simulink model "eq_sim"  (Simulink 6.0)
settings: Solver=VariableStepDiscrete  SolverMode=SingleTasking  StartTime=0.0  StopTime=10  RelTol=1e-3
StopFcn:
  | % Call to callback function in eq_initmask
  | if exist('taps','var')
  | eq_initmask([gcs '/Initial Settings'],'plotCostTrajectory',taps,tapsRef,eq);
  | end
model workspace: external: M-Code (data not in the file)
values from neighbouring files (symbols this model uses):
  eq = varargin{3}    [eq_initmask.m]
undefined symbols (not defined in the file or in its folder): eq_getopt, eq_mmseconverg, Fs, slcm
libraries: simulink x8, dspsigops x7, dspsrcs4 x6, dspsnks4 x6, commsink2 x5, dspsigattribs x5, commdigbbndam2 x3, commeq2 x2, dspindex x2, dspbuff3 x2, commchan2 x1, dsparch4 x1
CloseFcn:
  | % Call to callback function in eq_initmask
  | eq_initmask([gcs '/Initial Settings'],'CloseFcn');
settings Model: Creator=arodrigu  LastModifiedBy=arodrigu
settings DataIOCC: LimitDataPoints=off  SaveOutput=off  SaveTime=off  SignalLoggingName=eqSigsOut
settings OptimizationCC: BooleanDataType=off  InlineInvariantSignals=off
settings DebuggingCC: CheckExecutionContextPreStartOutputMsg=on  CheckExecutionContextRuntimeOutputMsg=on  SolverPrmCheckMsg=none  InheritedTsInSrcMsg=none
settings HardwareCC: TargetUnknown=on
settings ModelReferenceCC: UpdateModelReferenceTargets=IfOutOfDate
settings CodeAppCC: PrefixModelToSubsysFcnNames=off

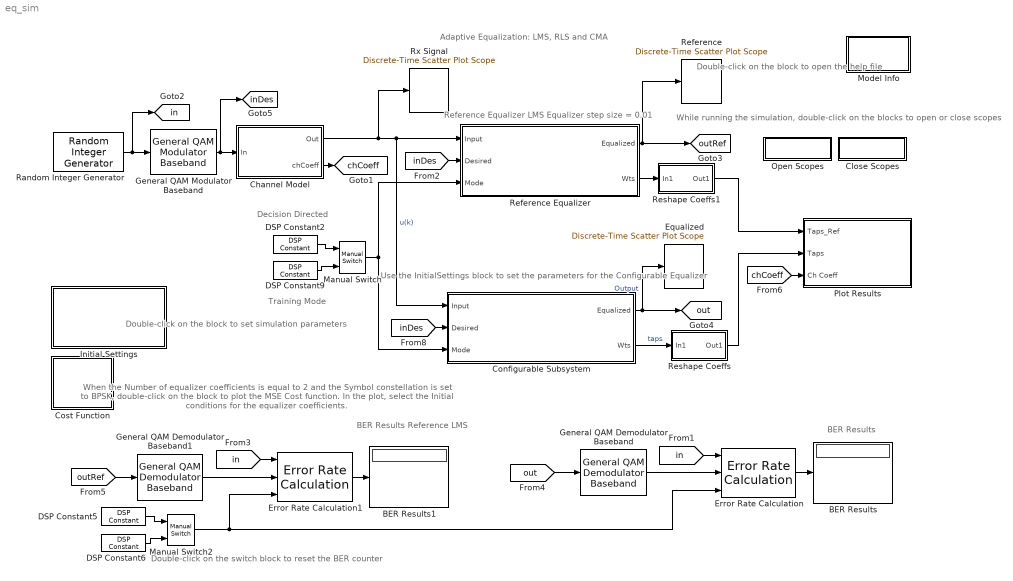
== system eq_sim ==
  note: Adaptive Equalization: LMS, RLS and CMA
  note: When the Number of equalizer coefficients is equal to 2 and the
      | Symbol constellation is set to BPSK, double-click on the block to plot
      | the MSE Cost function. In the plot, select the Initial conditions
      | for the equalizer coefficients.
  note: Double-click on the block
      | to set simulation parameters
  note: While running the simulation,
      | double-click on the blocks
      | to open or close scopes
  note: Training Mode
  note: Decision Directed
  note: BER Results
      | Reference LMS
  note: Double-click on the switch block
      | to reset the BER counter
  note: Reference Equalizer
      | LMS Equalizer
      | step size = 0.01
  note: BER Results
  note: Double-click on the block
      | to open the help file
  note: Use the InitialSettings block
      | to set the parameters for
      | the Configurable Equalizer
  BER Results : Display
  BER Results1 : Display
  Channel Model : Subsystem  PropExecContextAcrossSSBoundary=on  mask(Channel Model){chCoeff=eq.chCoeff, snrdB=eq.snrdB}
      mask prompts: chCoeff "Channel Coefficients:"; snrdB "SNR (in dB):"
      mask init:
      | chCoeff_fdB = 10*log10(abs(abs(fftshift(fft(chCoeff,256)))));
      | sigmaN2 = 10^(-snrdB/10);
      mask Display: plot([-pi:pi/128:(pi-pi/128)],chCoeff_fdB);
  Close Scopes : Subsystem  PropExecContextAcrossSSBoundary=on
      settings: OpenFcn=|
      | str1 = 'Plot Results';
      |         str2 = 'MSE Convergency Plot';
      |         str3 = 'Equalizer Response';
      |         str4 = 'Equalizer Taps - Real';
      |         str5 = 'Equalizer Taps - Imag';
      |         str6 = 'Rx Signal';
      |         str7 = 'Reference';
      |         str8 = 'Equalized';
      | 
      |         sdspfscope2([],[],[],'ScopeUpdate',[bdroot '/' str1 '/' str2 ],'CloseFig');
      |         sdspfscope2([],[],[],'ScopeUpdate',[bdroot '/' str1 '/' str3 ],'CloseFig');
      |         sdspfscope2([],[],[],'ScopeUpdate',[bdroot '/' str1 '/' str4 ],'CloseFig');
      |         sdspfscope2([],[],[],'ScopeUpdate',[bdroot '/' str1 '/' str5 ],'CloseFig');
      | 
      |         sdspfscope2([],[],[],'ScopeUpdate',[bdroot '/' str6 ],'CloseFig');
      |         sdspfscope2([],[],[],'ScopeUpdate',[bdroot '/' str7 ],'CloseFig');
      |         sdspfscope2([],[],[],'ScopeUpdate',[bdroot '/' str8 ],'CloseFig');
      mask Display: disp('Close Scopes');
  Configurable Subsystem : Subsystem  BlockChoice="RLS Linear  Equalizer"  PropExecContextAcrossSSBoundary=on
      link override CMA Equalizer: nTaps=eq.numTaps  sigConst=eq.const  delay=eq.delta_opt+1  stepSize=eq.stepSize  leakage=eq.leakage  initWeights=eq.ic
      link override LMS Linear  Equalizer: nTaps=eq.numTaps  sigConst=eq.const  delay=eq.delta_opt+1  stepSize=eq.stepSize  leakage=eq.leakage  initWeights=eq.ic
      link override Normalized LMS  Linear Equalizer: nTaps=eq.numTaps  sigConst=eq.const  delay=eq.delta_opt+1  stepSize=eq.stepSize  leakage=eq.leakage  bias=eq.norm  initWeights=eq.ic
      link override RLS Linear  Equalizer: nTaps=eq.numTaps  sigConst=eq.const  delay=eq.delta_opt+1  lambda=eq.lambda  invCorr=eq.icCorr  initWeights=eq.ic
      link override Sign LMS Linear  Equalizer: nTaps=eq.numTaps  sigConst=eq.const  delay=eq.delta_opt+1  stepSize=eq.stepSize  leakage=eq.leakage  initWeights=eq.ic
      link override Variable Step LMS  Linear Equalizer: nTaps=eq.numTaps  sigConst=eq.const  delay=eq.delta_opt+1  initMu=eq.muParIni  incMu=eq.muParStep  minMu=eq.muParMin  maxMu=eq.muParMax  leakage=eq.leakage  initWeights=eq.ic
      settings: AttributesFormatString=%<BlockChoice>  TemplateBlock=eq_lib/Configurable Subsystem  MemberBlocks="CMA Equalizer,LMS Linear  Equalizer,Normalized LMS  Linear Equalizer,RLS Linear  Equalizer,Sign LMS Linear  Equalizer,Variable Step LMS  Linear Equalizer"
      mask Display: disp(get_param(gcb,'BlockChoice'))
  Cost Function : Subsystem  PropExecContextAcrossSSBoundary=on
      settings: OpenFcn=eq_initmask([gcs '/Initial Settings'],'plotCostFcn');
      mask Type: Plot Cost Function
      mask Help: eval('commdemohelp;');
      mask Display: disp('Plot\nCost\nFunction');
  DSP Constant2 : dspsrcs4/DSP Constant  Value=0  SampleMode=Discrete  discreteOutput=Frame-based  continuousOutput=Sample-based  sampTime=1  framePeriod=1  dataType=Inherit from 'Constant value'  isSigned=on  wordLen=16  udDataType=sfix(16)  fracBitsMode=Best precision  numFracBits=15  InterpretAs1D=off  Ts=1  FramebasedOutput=on
      settings: AttributesFormatString=\n\n\n\n
  DSP Constant5 : dspsrcs4/DSP Constant  Value=0  SampleMode=Discrete  discreteOutput=Frame-based  continuousOutput=Sample-based  sampTime=1  framePeriod=1  dataType=Inherit from 'Constant value'  isSigned=on  wordLen=16  udDataType=sfix(16)  fracBitsMode=Best precision  numFracBits=15  InterpretAs1D=off  Ts=1  FramebasedOutput=on
      settings: AttributesFormatString=\n\n\n\n
  DSP Constant6 : dspsrcs4/DSP Constant  Value=1  SampleMode=Discrete  discreteOutput=Frame-based  continuousOutput=Sample-based  sampTime=1  framePeriod=1  dataType=Inherit from 'Constant value'  isSigned=on  wordLen=16  udDataType=sfix(16)  fracBitsMode=Best precision  numFracBits=15  InterpretAs1D=off  Ts=1  FramebasedOutput=on
      settings: AttributesFormatString=\n\n\n\n
  DSP Constant9 : dspsrcs4/DSP Constant  Value=1  SampleMode=Discrete  discreteOutput=Frame-based  continuousOutput=Sample-based  sampTime=1  framePeriod=1  dataType=Inherit from 'Constant value'  isSigned=on  wordLen=16  udDataType=sfix(16)  fracBitsMode=Best precision  numFracBits=15  InterpretAs1D=off  Ts=1  FramebasedOutput=on
      settings: AttributesFormatString=\n\n\n\n
  Equalized : commsink2/Discrete-Time Scatter Plot Scope  Tag=ScatterPlot  sampPerSymb=1  offsetEye=0  numTraces=200  numNewFrames=100  LineMarkers=.  LineColors=b  fading=on  render=on  AxisGrid=on  xMin=-1.6655405290464  xMax=1.67983399922447  yMin=-1.69487919740261  yMax=1.65049533086826  inphaseLabel=""  quadratureLabel=""  openScopeAtSimStart=on  FrameNumber=off  FigPos=[700 100 197 197]  figTitle=""  numLinesMax=50  block_type_=scatter
  Error Rate Calculation : commsink2/Error Rate Calculation  N=eq.delta_opt+1  st_delay=0  cp_mode=Entire frame  subframe=[]  PMode=Port  WsName=ErrorVec  RsMode2=on  stop=off  numErr=100  maxBits=1e6
  Error Rate Calculation1 : commsink2/Error Rate Calculation  N=eq.delta_opt+1  st_delay=0  cp_mode=Entire frame  subframe=[]  PMode=Port  WsName=ErrorVec  RsMode2=on  stop=off  numErr=100  maxBits=1e6
  General QAM Demodulator Baseband : commdigbbndam2/General QAM Demodulator Baseband  SigCon=eq.const  numSamp=1
  General QAM Demodulator Baseband1 : commdigbbndam2/General QAM Demodulator Baseband  SigCon=eq.const  numSamp=1
  General QAM Modulator Baseband : commdigbbndam2/General QAM Modulator Baseband  SigCon=eq.const  numSamp=1
  Initial Settings : Subsystem  PropExecContextAcrossSSBoundary=on  mask(Adaptive Equalization Example){chCoeff=[1 0.5 0.3], snrdB=40, numTaps=2, eqAlg=RLS - Recursive Least-Squares, symConst=BPSK, symConstCMA=BPSK, Mconst=16, stepSize=0.1, normalBias=1e-3, leakage=1, muParIni=0.1, muParStep=0.01, muParMax=0.3, muParMin=1e-4, lambdaPar=0.9, icCorr=100, icCoeff=[0.62379    -0.17516], displayChk=off}
      mask prompts: chCoeff "FIR Channel coefficients:"; snrdB "SNR (in dB):"; numTaps "Number of equalizer coefficients:"; eqAlg "Equalization Algorithm"; symConst "Symbol Constellation"; symConstCMA "Symbol Constellation"; Mconst "Number of points in constellation:"; stepSize "Step-size:"; normalBias "Normalization bias:"; leakage "Leakage factor:"; muParIni "Initial Step-size parameter:"; muParStep "Increment value of Step-size parameter:"; muParMax "Maximum Step-size parameter:"; muParMin "Minimum Step-size parameter:"; lambdaPar "Forgetting factor (lambda):"; icCorr "Initial conditions for inverse correlation matrix:"; icCoeff "Initial conditions for equalizer coefficients:"; displayChk "Display optimum values in the workspace"
      mask help:
      | Compare the performance of different T-space linear equalizers with a reference equalizer.
      |
      | Use the following mask to select the different parameters for the simulation.
      mask init:
      | eStr = eq_initmask(gcb,'init');
      | 		
      | if ~isempty(eStr.emsg)
      | 	errordlg(eStr.emsg, 'Equalizer Demo', 'replace');
      | end
      | 
      | if ~isempty(eStr.emsg_w) 
      | 	warndlg(eStr.emsg_w, 'Equalizer Demo', 'replace');
      | end
      mask Help: eval('commdemohelp;');
      mask StyleString: edit,edit,edit,popup(LMS - Least-Mean-Square|Sign LMS|NLMS - Normalized LMS|VSLMS - Variable Step-size LMS|RLS - Recursive Least-Squares|CMA - Constant Modulus Algorithm),popup(BPSK|QPSK|M-PSK|M-QAM),popup(BPSK|QPSK|M-PSK),edit,edit,edit,edit,edit,edit,edit,edit,edit,edit,edit,checkbox
      mask CallbackString: ||eq_initmask(gcb,'cbNumTaps');|eq_initmask(gcb,'cbEqAlg');|eq_initmask(gcb,'cbSymConst');|eq_initmask(gcb,'cbSymConstCMA');|eq_initmask(gcb,'cbMconst');|||||||||||
      mask Display: disp('Initial Settings')
  Manual Switch : simulink/Signal Routing/Manual Switch  sw=0  action=0
  Manual Switch2 : simulink/Signal Routing/Manual Switch  sw=1  action=0
  Model Info : Subsystem  LoadFcn=slcm LoadBlock;  InitFcn=slcm('UpdateAllCMBlocksInThisModelInit')  PropExecContextAcrossSSBoundary=on  mask(CMBlock){InitialSaveTempField=, InitialBlockCM=none, BlockCM=none, Frame=on, SaveTempField=, DisplayStringWithTags=Info, MaskDisplayString=Info, HorizontalTextAlignment=Center, LeftAlignmentValue=0.5, SourceBlockDiagram=eq_sim, TagMaxNumber=20, CMTag1=, CMTag2=, CMTag3=, CMTag4=, CMTag5=, CMTag6=, CMTag7=, CMTag8=, CMTag9=, CMTag10=, CMTag11=, CMTag12=, CMTag13=, CMTag14=, CMTag15=, CMTag16=, CMTag17=, CMTag18=, CMTag19=, CMTag20=}
      mask help: This block allows revision control information to be displayed within the model.
      settings: CopyFcn=slcm CopyBlock;  DeleteFcn=slcm Cancel;  PostSaveFcn=slcm('UpdateAllCMBlocksInThisModel')  NameChangeFcn=slcm Rename;  OpenFcn=commdemohelp;
      mask Display: text(str2num(LeftAlignmentValue), 0.5, MaskDisplayString, 'HorizontalAlignment', HorizontalTextAlignment)
  Open Scopes : Subsystem  PropExecContextAcrossSSBoundary=on
      settings: OpenFcn=|
      | str1 = 'Plot Results';
      |         str2 = 'MSE Convergency Plot';
      |         str3 = 'Equalizer Response';
      |         str4 = 'Equalizer Taps - Real';
      |         str5 = 'Equalizer Taps - Imag';
      |         str6 = 'Rx Signal';
      |         str7 = 'Reference';
      |         str8 = 'Equalized';
      | 
      |         sdspfscope2([],[],[],'ScopeUpdate',[bdroot '/' str1 '/' str2 ],'OpenFig');
      |         sdspfscope2([],[],[],'ScopeUpdate',[bdroot '/' str1 '/' str3 ],'OpenFig');
      |         sdspfscope2([],[],[],'ScopeUpdate',[bdroot '/' str1 '/' str4 ],'OpenFig');
      |         sdspfscope2([],[],[],'ScopeUpdate',[bdroot '/' str1 '/' str5 ],'OpenFig');
      | 
      |         sdspfscope2([],[],[],'ScopeUpdate',[bdroot '/' str6 ],'OpenFig');
      |         sdspfscope2([],[],[],'ScopeUpdate',[bdroot '/' str7 ],'OpenFig');
      |         sdspfscope2([],[],[],'ScopeUpdate',[bdroot '/' str8 ],'OpenFig');
      mask Type: Open Scopes
      mask Display: disp('Open Scopes');
  Plot Results : Subsystem  PropExecContextAcrossSSBoundary=on
      mask Display:
      | disp('Plot Results')
      | port_label('input',1,'tapsRef')
      | port_label('input',2,'taps')
      | port_label('input',3,'chCoeff')
  Random Integer Generator : commrandsrc2/Random Integer Generator  mul=eq.MConst  seed=12345  Ts=1/100  frameBased=on  sampPerFrame=100  orient=off
  Reference : commsink2/Discrete-Time Scatter Plot Scope  Tag=ScatterPlot  sampPerSymb=1  offsetEye=0  numTraces=200  numNewFrames=100  LineMarkers=.  LineColors=b  fading=on  render=on  AxisGrid=on  xMin=-1.6655405290464  xMax=1.67983399922447  yMin=-1.69487919740261  yMax=1.65049533086826  inphaseLabel=""  quadratureLabel=""  openScopeAtSimStart=on  FrameNumber=off  FigPos=[700 350 197 197]  figTitle=""  numLinesMax=50  block_type_=scatter
  Reference Equalizer : Subsystem  BlockChoice="LMS Linear  Equalizer"  PropExecContextAcrossSSBoundary=on
      link override CMA Equalizer: nTaps=eq.numTaps  sigConst=eq.const  delay=eq.delta_opt+1  stepSize=eq.stepSize  leakage=eq.leakage  initWeights=eq.ic
      link override LMS Linear  Equalizer: nTaps=eq.numTaps  sigConst=eq.const  delay=eq.delta_opt+1  stepSize=0.01  leakage=1  initWeights=eq.ic
      link override Normalized LMS  Linear Equalizer: nTaps=eq.numTaps  sigConst=eq.const  delay=eq.delta_opt+1  stepSize=eq.stepSize  leakage=eq.leakage  bias=eq.norm  initWeights=eq.ic
      link override RLS Linear  Equalizer: nTaps=eq.numTaps  sigConst=eq.const  delay=eq.delta_opt+1  lambda=eq.lambda  invCorr=eq.icCorr  initWeights=eq.ic
      link override Sign LMS Linear  Equalizer: nTaps=eq.numTaps  sigConst=eq.const  delay=eq.delta_opt+1  stepSize=eq.stepSize  leakage=eq.leakage  initWeights=eq.ic
      link override Variable Step LMS  Linear Equalizer: nTaps=eq.numTaps  sigConst=eq.const  delay=eq.delta_opt+1  initMu=eq.muParIni  incMu=eq.muParStep  minMu=eq.muParMin  maxMu=eq.muParMax  leakage=eq.leakage  initWeights=eq.ic
      settings: AttributesFormatString=%<BlockChoice>  TemplateBlock=eq_lib/Configurable Subsystem  MemberBlocks="CMA Equalizer,LMS Linear  Equalizer,Normalized LMS  Linear Equalizer,RLS Linear  Equalizer,Sign LMS Linear  Equalizer,Variable Step LMS  Linear Equalizer"
      mask Display: disp(get_param(gcb,'BlockChoice'))
  Reshape Coeffs : Subsystem  PropExecContextAcrossSSBoundary=on
  Reshape Coeffs1 : Subsystem  PropExecContextAcrossSSBoundary=on
  Rx Signal : commsink2/Discrete-Time Scatter Plot Scope  Tag=ScatterPlot  sampPerSymb=1  offsetEye=0  numTraces=200  numNewFrames=100  LineMarkers=.  LineColors=b  fading=on  render=on  AxisGrid=on  xMin=-1.5  xMax=1.5  yMin=-1.5  yMax=1.5  inphaseLabel=.  quadratureLabel=""  openScopeAtSimStart=on  FrameNumber=off  FigPos=[700 600 197 197]  figTitle=""  numLinesMax=50  block_type_=scatter
  tag scope: chCoeff=global, in=global, inDes=global, out=global, outRef=global
  wires:
  Channel Model/1(Out) -> Reference Equalizer/1(Input), Configurable Subsystem/1(Input), Rx Signal/1  "u(k)"
  Random Integer Generator/1 -> [in], General QAM Modulator Baseband/1
  [inDes] -> Reference Equalizer/2(Desired)
  Manual Switch/1 -> Reference Equalizer/3(Mode), Configurable Subsystem/3(Mode)
  Configurable Subsystem/2(Wts) -> Reshape Coeffs/1(In1)  "taps"
  [chCoeff] -> Plot Results/3(Ch Coeff)
  Reshape Coeffs/1(Out1) -> Plot Results/2(Taps)
  DSP Constant2/1 -> Manual Switch/1
  DSP Constant9/1 -> Manual Switch/2
  [inDes] -> Configurable Subsystem/2(Desired)
  Reference Equalizer/2(Wts) -> Reshape Coeffs1/1(In1)
  Reshape Coeffs1/1(Out1) -> Plot Results/1(Taps_Ref)
  Reference Equalizer/1(Equalized) -> Reference/1, [outRef]
  Configurable Subsystem/1(Equalized) -> [out], Equalized/1  "Output"
  [in] -> Error Rate Calculation1/1
  Error Rate Calculation1/1 -> BER Results1/1
  [outRef] -> General QAM Demodulator Baseband1/1
  Manual Switch2/1 -> Error Rate Calculation1/3, Error Rate Calculation/3
  DSP Constant5/1 -> Manual Switch2/1
  DSP Constant6/1 -> Manual Switch2/2
  General QAM Demodulator Baseband1/1 -> Error Rate Calculation1/2
  Channel Model/2(chCoeff) -> [chCoeff]
  [in] -> Error Rate Calculation/1
  Error Rate Calculation/1 -> BER Results/1
  [out] -> General QAM Demodulator Baseband/1
  General QAM Demodulator Baseband/1 -> Error Rate Calculation/2
  General QAM Modulator Baseband/1 -> Channel Model/1(In), [inDes]

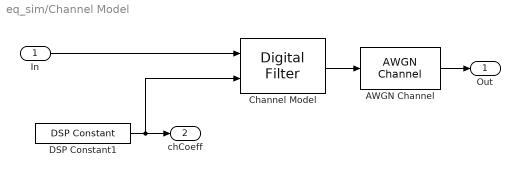
== system eq_sim/Channel Model ==
  In : Inport  LatchInput=off
  AWGN Channel : commchan2/AWGN Channel  seed=1237  noiseMode="Signal to noise ratio  (SNR)"  EbNodB=10  EsNodB=10  SNRdB=snrdB  bitsPerSym=1  Ps=1  Tsym=1  variance=sigmaN2
  Channel Model : dsparch4/Digital Filter  TypePopup=FIR (all zeros)  IIRFiltStruct=Direct form II transposed  AllPoleFiltStruct=Direct form  FIRFiltStruct=Direct form transposed  CoeffSource=Input port(s)  NumCoeffs=chCoeff  DenCoeffs=[1 0.1]  BiQuadCoeffs=[1 0.3 0.4 1 0.1 0.2]  LatticeCoeffs=[0.2 0.4]  denIgnore=on  FiltPerSampPopup=One filter per frame  IC=0  ICnum=0  ICden=0  roundingMode=Floor  overflowMode=off
  DSP Constant1 : dspsrcs4/DSP Constant  Value=eq.chCoeff  SampleMode=Discrete  discreteOutput=Frame-based  continuousOutput=Sample-based  sampTime=1  framePeriod=1  dataType=Inherit from 'Constant value'  wordLen=16  udDataType=sfix(16)  fracBitsMode=Best precision  numFracBits=15  InterpretAs1D=off  Ts=1  FramebasedOutput=on
  Out : Outport
  chCoeff : Outport  Port=2
  wires:
  Channel Model/1 -> AWGN Channel/1
  In/1 -> Channel Model/1
  AWGN Channel/1 -> Out/1
  DSP Constant1/1 -> Channel Model/2, chCoeff/1

== system eq_sim/Close Scopes ==
  note: This subsystem is empty

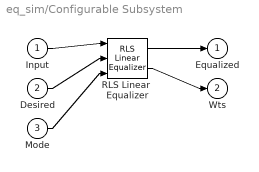
== system eq_sim/Configurable Subsystem ==
  Input : Inport  LatchInput=off
  Desired : Inport  Port=2  LatchInput=off
  Mode : Inport  Port=3  LatchInput=off
  RLS Linear  Equalizer : commeq2/RLS Linear  Equalizer  nTaps=eq.numTaps  nSamp=1  sigConst=eq.const  delay=eq.delta_opt+1  lambda=eq.lambda  invCorr=eq.icCorr  initWeights=eq.ic  mode=on  outErr=off  outWeights=on
  Equalized : Outport
  Wts : Outport  Port=2
  wires:
  Input/1 -> RLS Linear  Equalizer/1
  Desired/1 -> RLS Linear  Equalizer/2
  Mode/1 -> RLS Linear  Equalizer/3
  RLS Linear  Equalizer/1 -> Equalized/1
  RLS Linear  Equalizer/2 -> Wts/1

== system eq_sim/Cost Function ==
  note: This subsystem is empty

== system eq_sim/Initial Settings ==
  note: This subsystem is empty

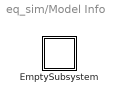
== system eq_sim/Model Info ==
  EmptySubsystem : Subsystem  PropExecContextAcrossSSBoundary=on

== system eq_sim/Open Scopes ==
  note: This subsystem is empty

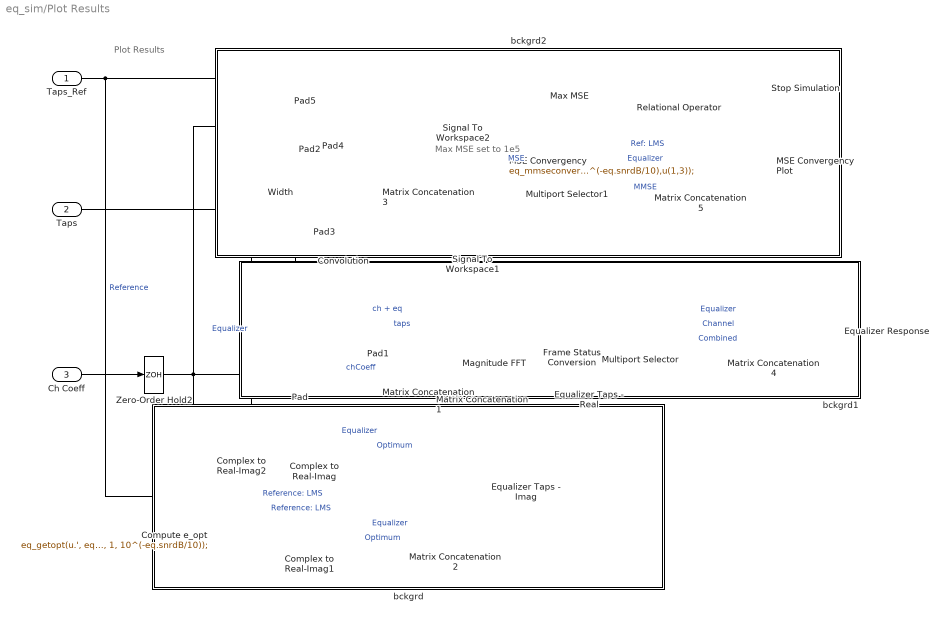
== system eq_sim/Plot Results ==
  note: Max MSE set to 1e5
  note: Plot Results
  Taps_Ref : Inport  LatchInput=off
  Taps : Inport  Port=2  LatchInput=off
  Ch Coeff : Inport  Port=3  LatchInput=off
  Complex to Real-Imag : ComplexToRealImag
  Complex to Real-Imag1 : ComplexToRealImag
  Complex to Real-Imag2 : ComplexToRealImag
  Compute e_opt : MATLABFcn  MATLABFcn=eq_getopt(u.', eq.numTaps, 1, 10^(-eq.snrdB/10));  OutputDimensions=[eq.numTaps 1]  OutputSignalType=complex  Output1D=off
  Convolution : dspsigops/Convolution  DialogController=dspDDGCreate  DialogControllerArgs=DataTag0  domain=Time  roundingMode=Floor  overflowMode=off
  Equalizer Response : dspsnks4/Vector Scope  ScopeProperties=off  Domain=Frequency  HorizSpan=1  DisplayProperties=on  AxisGrid=on  Memory=off  FrameNumber=off  AxisLegend=on  AxisZoom=off  OpenScopeAtSimStart=on  OpenScopeImmediately=off  FigPos=[280 140 403 256]  AxisProperties=off  XUnits=Hertz  XRange=[-Fs/2...Fs/2]  InheritXIncr=on  XIncr=1  XLabel=Time  YUnits=dB  YLabel=Magnitude  LineProperties=off  LineColors=[0 0 1]|[1 0 0]|[0 0 0]
      settings: AttributesFormatString=\n\n  YMin=-26.3159423323946  YMax=13.658558955862
  Equalizer Taps - Imag : dspsnks4/Vector Scope  ScopeProperties=off  Domain=User-defined  HorizSpan=1  DisplayProperties=off  AxisGrid=on  Memory=off  FrameNumber=off  AxisLegend=on  AxisZoom=off  OpenScopeAtSimStart=on  OpenScopeImmediately=off  FigPos=[0 140 266 255]  AxisProperties=off  XUnits=Hertz  XRange=[0...Fs/2]  InheritXIncr=off  XIncr=1  XLabel=Filter Coefficients  YUnits=dB  YLabel=Coefficients - Imag part  LineProperties=off  LineStyles=|--  LineMarkers=o|x|.  LineColors=[1 0 0]|[0 0 1]
      settings: AttributesFormatString=\n\n  YMin=-1  YMax=1
  Equalizer Taps - Real : dspsnks4/Vector Scope  ScopeProperties=off  Domain=User-defined  HorizSpan=1  DisplayProperties=on  AxisGrid=on  Memory=off  FrameNumber=off  AxisLegend=on  AxisZoom=off  OpenScopeAtSimStart=on  OpenScopeImmediately=off  FigPos=[0 446 267 255]  AxisProperties=off  XUnits=Hertz  XRange=[0...Fs/2]  InheritXIncr=off  XIncr=1  XLabel=Filter Coefficients  YUnits=dB  YLabel=Coefficients - Real Part  LineProperties=off  LineStyles=||--  LineMarkers=o|x|.  LineColors=[1 0 0]|[0 0 1]
      settings: AttributesFormatString=\n\n  YMin=-1  YMax=1
  Frame Status Conversion : dspsigattribs/Frame Status Conversion  growRefPort=off  outframe=Frame-based
  MSE Convergency : MATLABFcn  MATLABFcn="eq_mmseconverg(u(:,[1 4]), u(:,2), eq.numTaps,  1, 10^(-eq.snrdB/10),u(1,3));"  OutputDimensions=[1 3]  OutputSignalType=real  Output1D=off
  MSE Convergency Plot : dspsnks4/Vector Scope  ScopeProperties=off  Domain=Time  HorizSpan=313  DisplayProperties=off  AxisGrid=on  Memory=off  FrameNumber=off  AxisLegend=on  AxisZoom=off  OpenScopeAtSimStart=on  OpenScopeImmediately=off  FigPos=[280 447 403 254]  AxisProperties=off  XUnits=Hertz  XRange=[0...Fs/2]  InheritXIncr=on  XIncr=1  XLabel=Time  YUnits=dB  YLabel=MSE Convergency  LineProperties=off  LineStyles=||--  LineMarkers=||None  LineColors=[1 0 0]|[0 0 1]|[0 0 0]
      settings: AttributesFormatString=\n\n  YMin=0  YMax=0.5
  Magnitude FFT : dspspect3/Magnitude FFT  mag_or_magsq=Magnitude squared  fftLenInherit=off  fftsize=256
  Matrix Concatenation{,1..2,4..5} (5 alike) : simulink/Math Operations/Matrix Concatenation  numInports=3  catMethod=Horizontal
  Matrix Concatenation3 : simulink/Math Operations/Matrix Concatenation  numInports=4  catMethod=Horizontal
  Max MSE : dspsrcs4/DSP Constant  Value=1e5  SampleMode=Discrete  discreteOutput=Frame-based  continuousOutput=Sample-based  sampTime=1  framePeriod=1  dataType=Inherit from 'Constant value'  isSigned=on  wordLen=16  udDataType=sfix(16)  fracBitsMode=Best precision  numFracBits=15  InterpretAs1D=off  Ts=1  FramebasedOutput=on
  Multiport Selector : dspindex/Multiport Selector  rowsOrCols=Columns  idxCellArray={2,3,1}  idxErrMode=Clip Index
      settings: AttributesFormatString=\n
  Multiport Selector1 : dspindex/Multiport Selector  rowsOrCols=Columns  idxCellArray={1,2,3}  idxErrMode=Clip Index
      settings: AttributesFormatString=\n
  Pad : dspsigops/Pad  padVal=0  padSigAt=End  padAlong=Columns  padNumOutRowsSpecMethod=User-specified  numOutRows=eq.numTaps+length(eq.chCoeff)-1  padNumOutColsSpecMethod=User-specified  numOutCols=1  trunc_flag=None
      settings: AttributesFormatString=\n
  Pad1 : dspsigops/Pad  padVal=0  padSigAt=End  padAlong=Columns  padNumOutRowsSpecMethod=User-specified  numOutRows=eq.numTaps+length(eq.chCoeff)-1  padNumOutColsSpecMethod=User-specified  numOutCols=1  trunc_flag=None
      settings: AttributesFormatString=\n
  Pad{2..5} (4 alike) : dspsigops/Pad  padVal=0  padSigAt=End  padAlong=Columns  padNumOutRowsSpecMethod=User-specified  numOutRows=25  padNumOutColsSpecMethod=User-specified  numOutCols=1  trunc_flag=None
      settings: AttributesFormatString=\n
  Relational Operator : RelationalOperator  Operator=<
  Signal To Workspace1 : dspsnks4/Signal To Workspace  VariableName=taps  FrameMode=Log frames separately (3-D array)
      settings: FixptAsFi=off
  Signal To Workspace2 : dspsnks4/Signal To Workspace  VariableName=tapsRef  FrameMode=Log frames separately (3-D array)
      settings: FixptAsFi=off
  Stop Simulation : Stop
  Width : Width
  Zero-Order Hold2 : ZeroOrderHold  SampleTime=1/100
  bckgrd : Subsystem  PropExecContextAcrossSSBoundary=on
      mask Display: disp('')
  bckgrd1 : Subsystem  PropExecContextAcrossSSBoundary=on
      mask Display: disp('')
  bckgrd2 : Subsystem  PropExecContextAcrossSSBoundary=on
      mask Display: disp('')
  wires:
  Max MSE/1 -> Relational Operator/1
  Relational Operator/1 -> Stop Simulation/1
  Matrix Concatenation5/1 -> MSE Convergency Plot/1
  Multiport Selector1/1 -> Relational Operator/2, Matrix Concatenation5/1  "Ref: LMS"
  Matrix Concatenation4/1 -> Equalizer Response/1
  Multiport Selector/3 -> Matrix Concatenation4/3  "Combined"
  Multiport Selector/2 -> Matrix Concatenation4/2  "Channel"
  Multiport Selector/1 -> Matrix Concatenation4/1  "Equalizer"
  Magnitude FFT/1 -> Frame Status Conversion/1
  Pad4/1 -> Matrix Concatenation3/3
  Width/1 -> Pad4/1
  Matrix Concatenation3/1 -> MSE Convergency/1
  Pad3/1 -> Signal To Workspace1/1, Matrix Concatenation3/4
  Pad2/1 -> Matrix Concatenation3/2
  Compute e_opt/1 -> Complex to Real-Imag1/1
  Matrix Concatenation2/1 -> Equalizer Taps - Imag/1
  Complex to Real-Imag1/2 -> Matrix Concatenation2/3  "Optimum"
  Complex to Real-Imag1/1 -> Matrix Concatenation1/3  "Optimum"
  Complex to Real-Imag/2 -> Matrix Concatenation2/2  "Equalizer"
  Complex to Real-Imag/1 -> Matrix Concatenation1/2  "Equalizer"
  Matrix Concatenation1/1 -> Equalizer Taps - Real/1
  Matrix Concatenation/1 -> Magnitude FFT/1
  Convolution/1 -> Matrix Concatenation/1  "ch + eq"
  Pad1/1 -> Matrix Concatenation/2  "taps"
  Ch Coeff/1 -> Zero-Order Hold2/1
  Pad/1 -> Matrix Concatenation/3  "chCoeff"
  Taps/1 -> Pad3/1, Pad1/1, Convolution/1, Complex to Real-Imag/1  "Equalizer"
  MSE Convergency/1 -> Multiport Selector1/1  "MSE"
  Taps_Ref/1 -> Pad5/1, Complex to Real-Imag2/1  "Reference"
  Complex to Real-Imag2/1 -> Matrix Concatenation1/1  "Reference: LMS"
  Complex to Real-Imag2/2 -> Matrix Concatenation2/1  "Reference: LMS"
  Pad5/1 -> Matrix Concatenation3/1, Signal To Workspace2/1
  Multiport Selector1/2 -> Matrix Concatenation5/2  "Equalizer"
  Multiport Selector1/3 -> Matrix Concatenation5/3  "MMSE"
  Zero-Order Hold2/1 -> Width/1, Pad2/1, Convolution/2, Pad/1, Compute e_opt/1
  Frame Status Conversion/1 -> Multiport Selector/1

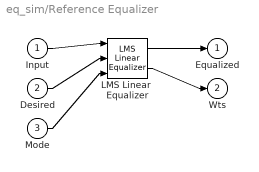
== system eq_sim/Reference Equalizer ==
  Input : Inport  LatchInput=off
  Desired : Inport  Port=2  LatchInput=off
  Mode : Inport  Port=3  LatchInput=off
  LMS Linear  Equalizer : commeq2/LMS Linear  Equalizer  nTaps=eq.numTaps  nSamp=1  sigConst=eq.const  delay=eq.delta_opt+1  stepSize=0.01  leakage=1  initWeights=eq.ic  mode=on  outErr=off  outWeights=on
  Equalized : Outport
  Wts : Outport  Port=2
  wires:
  Input/1 -> LMS Linear  Equalizer/1
  Desired/1 -> LMS Linear  Equalizer/2
  Mode/1 -> LMS Linear  Equalizer/3
  LMS Linear  Equalizer/1 -> Equalized/1
  LMS Linear  Equalizer/2 -> Wts/1

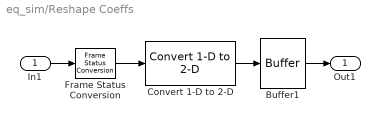
== system eq_sim/Reshape Coeffs ==
  In1 : Inport  LatchInput=off
  Buffer1 : dspbuff3/Buffer  N=eq.numTaps  V=0  ic=0
  Convert 1-D to 2-D : dspsigattribs/Convert 1-D to 2-D  M=eq.numTaps*100  N=1  frameBasedOut=on
  Frame Status Conversion : dspsigattribs/Frame Status Conversion  growRefPort=off  outframe=Frame-based
  Out1 : Outport
  wires:
  Frame Status Conversion/1 -> Convert 1-D to 2-D/1
  Convert 1-D to 2-D/1 -> Buffer1/1
  Buffer1/1 -> Out1/1
  In1/1 -> Frame Status Conversion/1

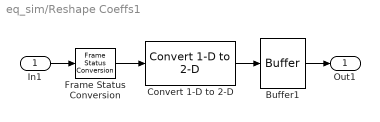
== system eq_sim/Reshape Coeffs1 ==
  In1 : Inport  LatchInput=off
  Buffer1 : dspbuff3/Buffer  N=eq.numTaps  V=0  ic=0
  Convert 1-D to 2-D : dspsigattribs/Convert 1-D to 2-D  M=eq.numTaps*100  N=1  frameBasedOut=on
  Frame Status Conversion : dspsigattribs/Frame Status Conversion  growRefPort=off  outframe=Frame-based
  Out1 : Outport
  wires:
  In1/1 -> Frame Status Conversion/1
  Buffer1/1 -> Out1/1
  Convert 1-D to 2-D/1 -> Buffer1/1
  Frame Status Conversion/1 -> Convert 1-D to 2-D/1

== system eq_sim/Model Info/EmptySubsystem ==

== system eq_sim/Plot Results/bckgrd ==
  note: This subsystem is empty

== system eq_sim/Plot Results/bckgrd1 ==
  note: This subsystem is empty

== system eq_sim/Plot Results/bckgrd2 ==
  note: This subsystem is empty
